simulink model "Vector_Control_Lib"  (R2021a)
settings: Solver=FixedStepDiscrete  StartTime=0.0  StopTime=1  FixedStep=Ts  RelTol=1e-3  EnableMultiTasking=on
values from neighbouring files (symbols this model uses):
  AccelTime = 1    [param.m]
  CurrentLSB = -1 * (1/ 0.1) * (3.3 / 2048)    (= -0.01611328125)    [param.m]
  DAC_ANALOG_MAX_0ch = 4    [param.m]
  DAC_ANALOG_MAX_1ch = 4    [param.m]
  DAC_PULSE_MAX = 4096    [param.m]
  DUTY_COUNTER_PERIOD_BASE = 2100    [param.m]
  EncoderLSB = 1/400    (= 0.0025)    [param.m]
  isEmbedded = swichSimulationMode('Emb')    [param.m]    (also in swichSimulationMode.m = boolean(0))
  Iu_ad_offset = 2020    [param.m]
  Iv_ad_offset = 2022    [param.m]
  Iw_ad_offset = 2020    [param.m]
  k_LPF = tauHPF / (tauHPF + Ts)    (= 0.999900009999)    [param.m]
  Ke = 4.50E-03    (= 0.0045)    [param.m]
  Ki_Ts = Ra / tauCurrent * Ts    (= 0.00075)    [param.m]
  Kp = La / tauCurrent    (= 0.009)    [param.m]
  La = 1.2e-3 * Ra    (= 0.0009)    [param.m]
  LockTime = 0.1    [param.m]
  omega_ref = 600    [param.m]
  Pn = 6    [param.m]
  Pz_ele = c2d(Ps_ele, Ts)    [param.m]
  Pz_mecha = c2d(Ps_mecha, Ts)    [param.m]
  TotalTime = LockTime + AccelTime    (= 1.1)    [param.m]
  Ts = 100e-6    (= 0.0001)    [param.m]
  Vdc = 10    [param.m]
libraries: simulink x21, arduinolib x4
settings Model: SILPILModeSetting=veronly  ExtModeTrigDuration=2  Creator=kuroda38  LastModifiedBy=kuroda38
settings OptimizationCC: EnhancedBackFolding=on  PassReuseOutputArgsAs=Individual arguments  ZeroExternalMemoryAtStartup=off  ZeroInternalMemoryAtStartup=off  MaxStackSize=64  OptimizeBlockOrder=speed  DifferentSizesBufferReuse=on  OptimizationCustomize=off  EfficientTunableParamExpr=on
settings DebuggingCC: ParameterTunabilityLossMsg=error
settings HardwareCC: ProdBitPerPointer=32  ProdBitPerSizeT=32  ProdBitPerPtrDiffT=32  ProdLargestAtomicInteger=Long  ProdLargestAtomicFloat=Double  ProdWordSize=32  ProdHWDeviceType=ARM Compatible->ARM Cortex  UseEmbeddedCoderFeatures=off  UseSimulinkCoderFeatures=off
settings SFSimCC: MATLABDynamicMemAlloc=off
settings RTWCC: SystemTargetFile=ert.tlc  HardwareBoard=Arduino Due  TemplateMakefile=ert_default_tmf  Toolchain=Arduino ARM  BuildConfiguration=Faster Runs
settings CodeAppCC: ForceParamTrailComments=on  IgnoreCustomStorageClasses=off  OperatorAnnotations=on  SimulinkDataObjDesc=on  SFDataObjDesc=on  InsertBlockDesc=on
settings ERTTargetCC: SupportContinuousTime=on  SupportNonInlinedSFcns=on  SupportVariableSizeSignals=on  ExtModeTransport=3  ExtModeStaticAlloc=on  ExtModeStaticAllocSize=24576  ExtModeMexFile=ext_xcp  ExtModeIntrfLevel=Level2 - Open

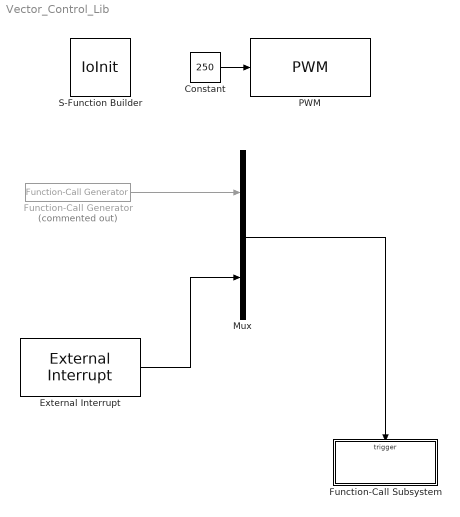
== system Vector_Control_Lib ==
  Constant : Constant  Value=250  OutDataTypeStr=uint8
  External Interrupt : arduinolib/External Interrupt  Pin=12  PullUp=off  Mode=RISING  InterruptSimulationInput=off
      settings: SourceProductBaseCode=ARDUINO
  Function-Call Generator : simulink/Ports & Subsystems/Function-Call Generator  Commented=on  sample_time=Ts  numberOfIterations=1  DisallowWideOutput=off
  Function-Call Subsystem : Subsystem  TreatAsAtomicUnit=on
  Mux : Mux  Inputs=2
  PWM : arduinolib/PWM  pinNumber=5  frequencyType=Specify  desiredFrequency=20000  achievableFrequency=20000
  S-Function Builder : S-Function  FunctionName=IoInit  SFunctionModules=IoInit_wrapper  SFunctionDeploymentMode=off  EnableBusSupport=off  mask(S-Function Builder){}
      mask help: Simulink:masks:SFunctionBuilder_MD
      mask init:
      | val = [[.9  0.75 0.75 1 1 .9 .9 1]',[1 1 0.75 0.75 .9 .9 1 .9]'];try , sys = get_param(gcb,'SfunBuilderFcnName');if isempty(sys), sys = get_param(gcb,'FunctionName'); end,catch, sys = get_param(gcb,'FunctionName'); end
      settings: CopyFcn=set_param(gcbh,'LinkStatus','none')  OpenFcn=sfunctionwizard(gcbh)
      mask Display:
      | plot(val(:,1),val(:,2))
      | disp(sys)
  wires:
  Constant/1 -> PWM/1
  Function-Call Generator/1 -> Mux/1
  Mux/1 -> Function-Call Subsystem/Trigger
  External Interrupt/1 -> Mux/2

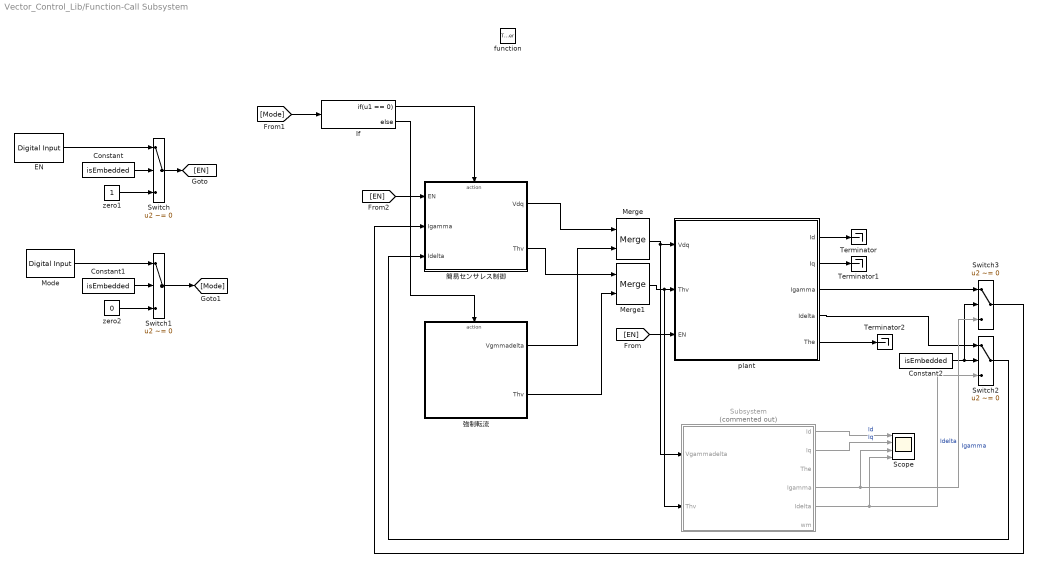
== system Vector_Control_Lib/Function-Call Subsystem ==
  function : TriggerPort  TriggerType=function-call  VariantControl=(inherit)
  Constant : Constant  Value=isEmbedded
  Constant1 : Constant  Value=isEmbedded
  Constant2 : Constant  Value=isEmbedded  OutDataTypeStr=uint8
  EN : arduinolib/Digital Input  pinNumber=7  mode=Default  Direction=input  SampleTime=-1  blockPlatform=arduino
  If : If  IfExpression=u1 == 0
  Merge : Merge
  Merge1 : Merge
  Mode : arduinolib/Digital Input  pinNumber=6  mode=Default  Direction=input  SampleTime=-1  blockPlatform=arduino
  Scope : Scope  NumInputPorts=4
  Subsystem : Subsystem  Commented=on
  Switch : Switch  Criteria=u2 ~= 0  OutDataTypeStr=uint16
  Switch1 : Switch  Criteria=u2 ~= 0  OutDataTypeStr=uint16
  Switch2 : Switch  Criteria=u2 ~= 0
  Switch3 : Switch  Criteria=u2 ~= 0
  Terminator : Terminator
  Terminator1 : Terminator
  Terminator2 : Terminator
  plant : Subsystem
  zero1 : Constant  OutDataTypeStr=uint16
  zero2 : Constant  Value=0  OutDataTypeStr=uint16
  強制転流 : Subsystem  TreatAsAtomicUnit=on
  簡易センサレス制御 : Subsystem  TreatAsAtomicUnit=on
  wires:
  [EN] -> plant/3(EN)
  Merge/1 -> plant/1(Vdq), Subsystem/1(Vgammadelta)
  Merge1/1 -> Subsystem/2(Thv), plant/2(Thv)
  If/1 -> 簡易センサレス制御/Action
  If/2 -> 強制転流/Action
  簡易センサレス制御/1(Vdq) -> Merge/1
  強制転流/1(Vgmmadelta) -> Merge/2
  簡易センサレス制御/2(Thv) -> Merge1/1
  強制転流/2(Thv) -> Merge1/2
  plant/1(Id) -> Terminator/1
  plant/2(Iq) -> Terminator1/1
  plant/5(The) -> Terminator2/1
  [EN] -> 簡易センサレス制御/1(EN)
  Constant/1 -> Switch/2
  Switch/1 -> [EN]
  EN/1 -> Switch/1
  zero1/1 -> Switch/3
  Constant1/1 -> Switch1/2
  zero2/1 -> Switch1/3
  Mode/1 -> Switch1/1
  Switch1/1 -> [Mode]
  [Mode] -> If/1
  Subsystem/1(Id) -> Scope/1  "Id"
  Subsystem/2(Iq) -> Scope/2  "Iq"
  plant/3(Igamma) -> Switch3/1
  plant/4(Idelta) -> Switch2/1
  Constant2/1 -> Switch3/2, Switch2/2
  Subsystem/4(Igamma) -> Scope/3, Switch3/3  "Igamma"
  Subsystem/5(Idelta) -> Scope/4, Switch2/3  "Idelta"
  Switch3/1 -> 簡易センサレス制御/2(Igamma)
  Switch2/1 -> 簡易センサレス制御/3(Idelta)

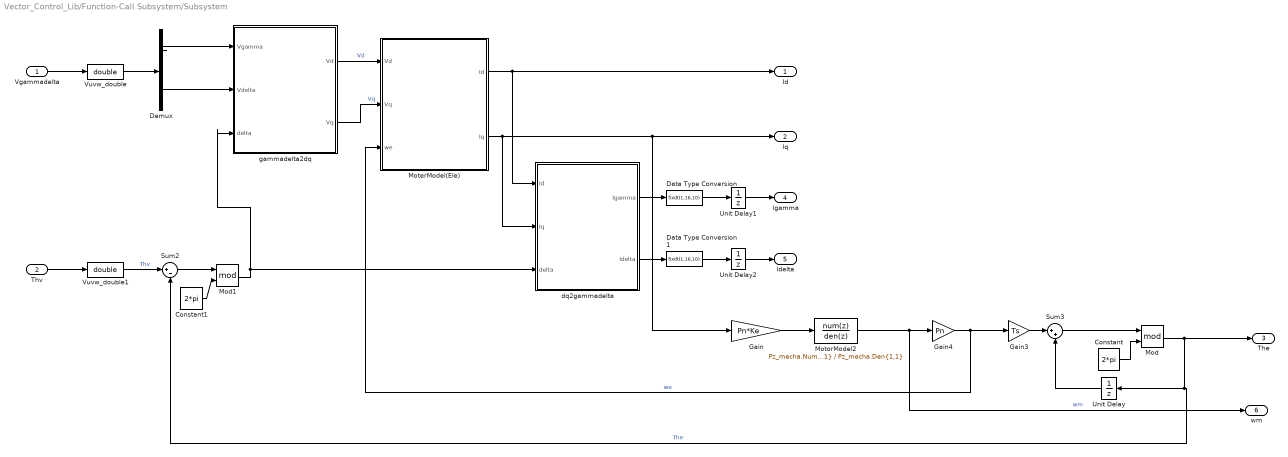
== system Vector_Control_Lib/Function-Call Subsystem/Subsystem ==
  Vgammadelta : Inport
  Thv : Inport  Port=2
  Constant : Constant  Value=2*pi
  Constant1 : Constant  Value=2*pi
  Data Type Conversion : DataTypeConversion  OutDataTypeStr=fixdt(1,16,10)
  Data Type Conversion1 : DataTypeConversion  OutDataTypeStr=fixdt(1,16,10)
  Demux : Demux  Outputs=2
  Gain : Gain  Gain=Pn*Ke
  Gain3 : Gain  Gain=Ts
  Gain4 : Gain  Gain=Pn
  Mod : Math  Operator=mod  SaturateOnIntegerOverflow=on
  Mod1 : Math  Operator=mod  SaturateOnIntegerOverflow=on
  MoterModel(Ele) : Subsystem
  MotorModel2 : DiscreteTransferFcn  Numerator=Pz_mecha.Num{1,1}  Denominator=Pz_mecha.Den{1,1}
  Sum2 : Sum  Inputs=|+-
  Sum3 : Sum  Inputs=|++
  Unit Delay : UnitDelay  SampleTime=-1  HasFrameUpgradeWarning=on
  Unit Delay1 : UnitDelay  SampleTime=-1  HasFrameUpgradeWarning=on
  Unit Delay2 : UnitDelay  SampleTime=-1  HasFrameUpgradeWarning=on
  Vuvw_double : DataTypeConversion  OutDataTypeStr=double
  Vuvw_double1 : DataTypeConversion  OutDataTypeStr=double
  dq2gammadelta : Subsystem
  gammadelta2dq : Subsystem
  Id : Outport
  Iq : Outport  Port=2
  The : Outport  Port=3
  Igamma : Outport  Port=4
  Idelta : Outport  Port=5
  wm : Outport  Port=6
  wires:
  Gain/1 -> MotorModel2/1
  MotorModel2/1 -> wm/1, Gain4/1  "wm"
  Vgammadelta/1 -> Vuvw_double/1
  Gain3/1 -> Sum3/1
  Vuvw_double/1 -> Demux/1
  Thv/1 -> Vuvw_double1/1
  Gain4/1 -> MoterModel(Ele)/3(we), Gain3/1  "we"
  Demux/1 -> gammadelta2dq/1(Vgamma)
  Demux/2 -> gammadelta2dq/2(Vdelta)
  MoterModel(Ele)/2(Iq) -> dq2gammadelta/2(Iq), Gain/1, Iq/1
  gammadelta2dq/1(Vd) -> MoterModel(Ele)/1(Vd)  "Vd"
  gammadelta2dq/2(Vq) -> MoterModel(Ele)/2(Vq)  "Vq"
  MoterModel(Ele)/1(Id) -> dq2gammadelta/1(Id), Id/1
  dq2gammadelta/1(Igamma) -> Data Type Conversion/1
  dq2gammadelta/2(Idelta) -> Data Type Conversion1/1
  Vuvw_double1/1 -> Sum2/1  "Thv"
  Constant/1 -> Mod/2
  Sum3/1 -> Mod/1
  Mod/1 -> Unit Delay/1, Sum2/2, The/1  "The"
  Unit Delay/1 -> Sum3/2
  Constant1/1 -> Mod1/2
  Sum2/1 -> Mod1/1
  Mod1/1 -> dq2gammadelta/3(delta), gammadelta2dq/3(delta)
  Data Type Conversion/1 -> Unit Delay1/1
  Unit Delay1/1 -> Igamma/1
  Data Type Conversion1/1 -> Unit Delay2/1
  Unit Delay2/1 -> Idelta/1

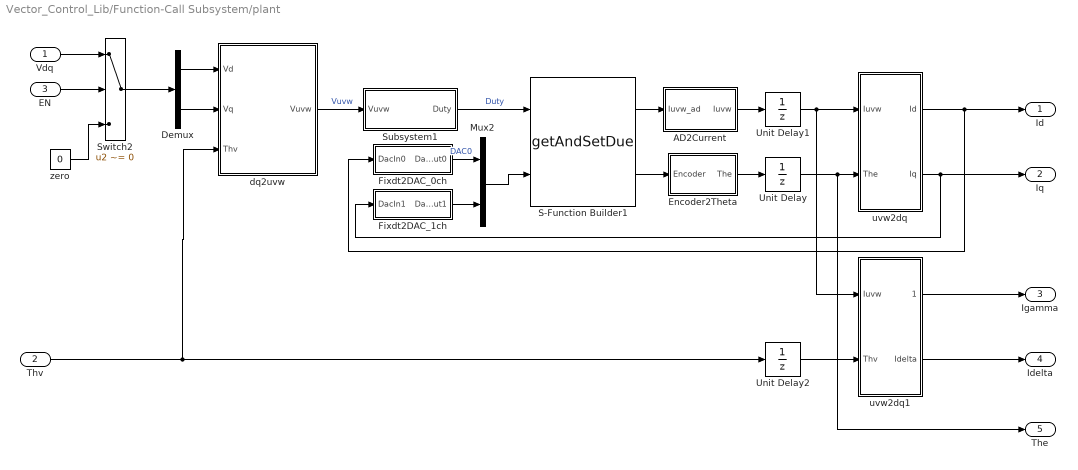
== system Vector_Control_Lib/Function-Call Subsystem/plant ==
  Vdq : Inport
  Thv : Inport  Port=2
  EN : Inport  Port=3
  AD2Current : Subsystem
  Demux : Demux  Outputs=2
  Encoder2Theta : Subsystem
  Fixdt2DAC_0ch : Subsystem
  Fixdt2DAC_1ch : Subsystem
  Mux2 : Mux  Inputs=2
  S-Function Builder1 : S-Function  FunctionName=getAndSetDue  SFunctionModules=getAndSetDue_wrapper  SFunctionDeploymentMode=off  EnableBusSupport=off  mask(S-Function Builder){}
      mask help: Simulink:masks:SFunctionBuilder_MD
      mask init: same as Vector_Control_Lib/S-Function Builder
      settings: CopyFcn=set_param(gcbh,'LinkStatus','none')  OpenFcn=sfunctionwizard(gcbh)
      mask Display:
      | plot(val(:,1),val(:,2))
      | disp(sys)
      | port_label('input',1,'Duty')
      | port_label('input',2,'DAC')
      | port_label('output',1,'Iuvw')
      | port_label('output',2,'Encoder')
  Subsystem1 : Subsystem
  Switch2 : Switch  Criteria=u2 ~= 0  OutDataTypeStr=fixdt(1,16,10)
  Unit Delay : UnitDelay  SampleTime=-1  HasFrameUpgradeWarning=on
  Unit Delay1 : UnitDelay  SampleTime=-1  HasFrameUpgradeWarning=on
  Unit Delay2 : UnitDelay  SampleTime=-1  HasFrameUpgradeWarning=on
  dq2uvw : Subsystem
  uvw2dq : Subsystem
  uvw2dq1 : Subsystem
  zero : Constant  Value=0  OutDataTypeStr=fixdt(1,16,10)
  Id : Outport
  Iq : Outport  Port=2
  Igamma : Outport  Port=3
  Idelta : Outport  Port=4
  The : Outport  Port=5
  wires:
  S-Function Builder1/2 -> Encoder2Theta/1(Encoder)
  AD2Current/1(Iuvw) -> Unit Delay1/1
  uvw2dq/2(Iq) -> Fixdt2DAC_1ch/1(DacIn1), Iq/1
  Fixdt2DAC_1ch/1(DacOut1) -> Mux2/2
  Fixdt2DAC_0ch/1(DacOut0) -> Mux2/1  "DAC0"
  Mux2/1 -> S-Function Builder1/2
  uvw2dq/1(Id) -> Id/1, Fixdt2DAC_0ch/1(DacIn0)
  Unit Delay/1 -> The/1, uvw2dq/2(The)
  dq2uvw/1(Vuvw) -> Subsystem1/1(Vuvw)  "Vuvw"
  Subsystem1/1(Duty) -> S-Function Builder1/1  "Duty"
  S-Function Builder1/1 -> AD2Current/1(Iuvw_ad)
  Unit Delay1/1 -> uvw2dq1/1(Iuvw), uvw2dq/1(Iuvw)
  Encoder2Theta/1(The) -> Unit Delay/1
  Thv/1 -> dq2uvw/3(Thv), Unit Delay2/1
  Vdq/1 -> Switch2/1
  EN/1 -> Switch2/2
  zero/1 -> Switch2/3
  Switch2/1 -> Demux/1
  Demux/1 -> dq2uvw/1(Vd)
  Demux/2 -> dq2uvw/2(Vq)
  uvw2dq1/1(Igamma) -> Igamma/1
  uvw2dq1/2(Idelta) -> Idelta/1
  Unit Delay2/1 -> uvw2dq1/2(Thv)

== system Vector_Control_Lib/Function-Call Subsystem/強制転流 ==
  Action Port : ActionPort  ActionPortLabel=else
  Mux : Mux  Inputs=2
  Omega_ref : Constant  Value=omega_ref  OutDataTypeStr=fixedTypeOmegaRef
  Vdelta : Constant  Value=2  OutDataTypeStr=fixdt(1,16,10)
  Vgamma : Constant  Value=0  OutDataTypeStr=fixdt(1,16,10)
  wv_integral : Subsystem
  Vgmmadelta : Outport
  Thv : Outport  Port=2
  wires:
  Vgamma/1 -> Mux/1
  Vdelta/1 -> Mux/2
  Mux/1 -> Vgmmadelta/1
  Omega_ref/1 -> wv_integral/1(wv_ref)  "Omega_ref"
  wv_integral/1(Thv) -> Thv/1  "Thv"

== system Vector_Control_Lib/Function-Call Subsystem/簡易センサレス制御 ==
  EN : Inport
  Igamma : Inport  Port=2
  Idelta : Inport  Port=3
  Action Port : ActionPort  ActionPortLabel=if(u1 == 0)
  Mux : Mux  Inputs=2
  VdeltaController : Subsystem
  Vgamma : Constant  Value=0  OutDataTypeStr=fixdt(1,16,10)
  wv_integral : Subsystem
  Vdq : Outport
  Thv : Outport  Port=2
  wires:
  Mux/1 -> Vdq/1
  EN/1 -> VdeltaController/1(EN)
  wv_integral/1(Thv) -> Thv/1  "Thv"
  VdeltaController/1(Omega_ref) -> wv_integral/1(wv_ref)  "Omega_ref"
  Vgamma/1 -> Mux/1
  Igamma/1 -> VdeltaController/2(Igamma)
  Idelta/1 -> VdeltaController/3(Idelta)
  VdeltaController/2(Vdelta) -> Mux/2

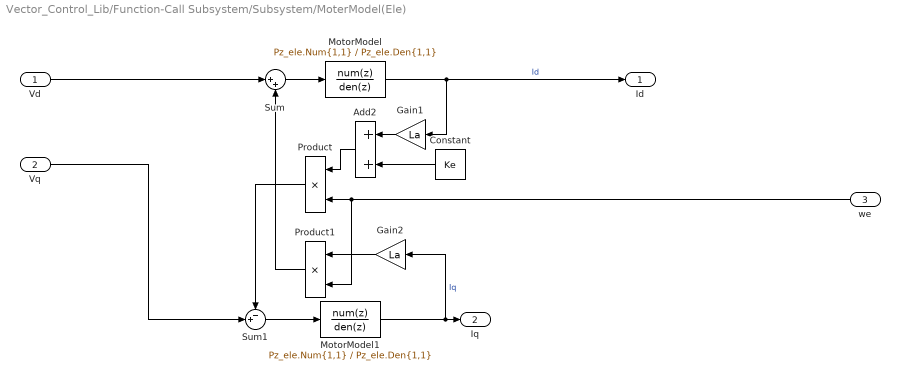
== system Vector_Control_Lib/Function-Call Subsystem/Subsystem/MoterModel(Ele) ==
  Vd : Inport
  Vq : Inport  Port=2
  we : Inport  Port=3
  Add2 : Sum
  Constant : Constant  Value=Ke
  Gain1 : Gain  Gain=La
  Gain2 : Gain  Gain=La
  MotorModel : DiscreteTransferFcn  Numerator=Pz_ele.Num{1,1}  Denominator=Pz_ele.Den{1,1}
  MotorModel1 : DiscreteTransferFcn  Numerator=Pz_ele.Num{1,1}  Denominator=Pz_ele.Den{1,1}
  Product : Product
  Product1 : Product
  Sum : Sum  Inputs=|++
  Sum1 : Sum  Inputs=-+|
  Id : Outport
  Iq : Outport  Port=2
  wires:
  we/1 -> Product1/2, Product/2
  MotorModel/1 -> Id/1, Gain1/1  "Id"
  Gain2/1 -> Product1/1
  Product/1 -> Sum1/1
  Constant/1 -> Add2/2
  Sum/1 -> MotorModel/1
  Gain1/1 -> Add2/1
  Product1/1 -> Sum/2
  Sum1/1 -> MotorModel1/1
  Add2/1 -> Product/1
  Vd/1 -> Sum/1
  Vq/1 -> Sum1/2
  MotorModel1/1 -> Gain2/1, Iq/1  "Iq"

== system Vector_Control_Lib/Function-Call Subsystem/Subsystem/dq2gammadelta ==
  Id : Inport
  Iq : Inport  Port=2
  delta : Inport  Port=3
  Add : Sum
  Add1 : Sum  Inputs=-+
  Cos2 : Trigonometry
  Cos3 : Trigonometry  Operator=cos
  Product{2..5} (4 alike) : Product
  Igamma : Outport
  Idelta : Outport  Port=2
  wires:
  delta/1 -> Cos2/1, Cos3/1
  Iq/1 -> Product5/1, Product3/1
  Product4/1 -> Add1/1
  Cos3/1 -> Product5/2, Product2/2
  Product3/1 -> Add/2
  Id/1 -> Product4/1, Product2/1
  Product2/1 -> Add/1
  Product5/1 -> Add1/2
  Cos2/1 -> Product3/2, Product4/2
  Add1/1 -> Idelta/1
  Add/1 -> Igamma/1

== system Vector_Control_Lib/Function-Call Subsystem/Subsystem/gammadelta2dq ==
  Vgamma : Inport
  Vdelta : Inport  Port=2
  delta : Inport  Port=3
  Add : Sum  Inputs=+-
  Add1 : Sum
  Cos2 : Trigonometry
  Cos3 : Trigonometry  Operator=cos
  Product{2..5} (4 alike) : Product
  Vd : Outport
  Vq : Outport  Port=2
  wires:
  delta/1 -> Cos2/1, Cos3/1
  Vdelta/1 -> Product5/1, Product3/1
  Product4/1 -> Add1/1
  Cos3/1 -> Product5/2, Product2/2
  Product3/1 -> Add/2
  Vgamma/1 -> Product4/1, Product2/1
  Product2/1 -> Add/1
  Product5/1 -> Add1/2
  Cos2/1 -> Product3/2, Product4/2
  Add1/1 -> Vq/1
  Add/1 -> Vd/1

== system Vector_Control_Lib/Function-Call Subsystem/plant/AD2Current ==
  Iuvw_ad : Inport
  Add : Sum  Inputs=+-  OutDataTypeStr=int16
  Add1 : Sum  Inputs=+-  OutDataTypeStr=int16
  Add2 : Sum  Inputs=+-  OutDataTypeStr=int16
  Constant : Constant  Value=Iu_ad_offset  OutDataTypeStr=uint16
  Constant1 : Constant  Value=Iv_ad_offset  OutDataTypeStr=uint16
  Constant2 : Constant  Value=CurrentLSB  OutDataTypeStr=fixdt(1,16)
  Constant3 : Constant  Value=Iw_ad_offset  OutDataTypeStr=uint16
  Demux : Demux  Outputs=3
  Mux : Mux  Inputs=3
  Product : Product  OutDataTypeStr=fixedTypeDqCurrent
  Iuvw : Outport
  wires:
  Demux/2 -> Add1/1
  Constant/1 -> Add/2
  Constant3/1 -> Add2/2
  Demux/3 -> Add2/1
  Constant1/1 -> Add1/2
  Demux/1 -> Add/1
  Add/1 -> Mux/1
  Add1/1 -> Mux/2
  Add2/1 -> Mux/3
  Product/1 -> Iuvw/1
  Constant2/1 -> Product/2
  Mux/1 -> Product/1
  Iuvw_ad/1 -> Demux/1

== system Vector_Control_Lib/Function-Call Subsystem/plant/Encoder2Theta ==
  Encoder : Inport
  Add : Sum  Inputs=+-  OutDataTypeStr=int16
  Constant : Constant  Value=36  OutDataTypeStr=uint16
  Constant1 : Constant  Value=EncoderLSB  OutDataTypeStr=fixedTypeMaxOne
  Constant2 : Constant  Value=Pn  OutDataTypeStr=ufixedTypeMaxTwenty
  Constant3 : Constant  Value=2*pi  OutDataTypeStr=ufixedTypeTwoPi
  Product : Product  OutDataTypeStr=ufixedTypeMaxOne
  Product1 : Product  OutDataTypeStr=fixdt(0,16,16)
  Product7 : Product  OutDataTypeStr=ufixedTypeTwoPi
  The : Outport
  wires:
  Encoder/1 -> Add/1
  Constant/1 -> Add/2
  Add/1 -> Product/1
  Constant1/1 -> Product/2
  Product/1 -> Product1/1
  Constant2/1 -> Product1/2
  Product1/1 -> Product7/1
  Product7/1 -> The/1
  Constant3/1 -> Product7/2

== system Vector_Control_Lib/Function-Call Subsystem/plant/Fixdt2DAC_0ch ==
  DacIn0 : Inport
  Add1 : Sum  OutDataTypeStr=fixdt(1,16,10)
  Constant4 : Constant  Value=DAC_ANALOG_MAX_0ch  OutDataTypeStr=fixdt(1,16)
  Constant7 : Constant  Value=(DAC_PULSE_MAX / 2 ) / DAC_ANALOG_MAX_0ch  OutDataTypeStr=fixdt(1,16)  LockScale=on
  Product1 : Product  OutDataTypeStr=uint16
  DacOut0 : Outport
  wires:
  Add1/1 -> Product1/1
  Constant7/1 -> Product1/2
  Constant4/1 -> Add1/2
  Product1/1 -> DacOut0/1
  DacIn0/1 -> Add1/1

== system Vector_Control_Lib/Function-Call Subsystem/plant/Fixdt2DAC_1ch ==
  DacIn1 : Inport
  Add1 : Sum  OutDataTypeStr=fixdt(1,16,10)
  Constant4 : Constant  Value=DAC_ANALOG_MAX_1ch  OutDataTypeStr=fixdt(1,16)
  Constant7 : Constant  Value=(DAC_PULSE_MAX / 2 ) / DAC_ANALOG_MAX_1ch  OutDataTypeStr=fixdt(1,16)  LockScale=on
  Product1 : Product  OutDataTypeStr=uint16
  DacOut1 : Outport
  wires:
  Add1/1 -> Product1/1
  Constant7/1 -> Product1/2
  Constant4/1 -> Add1/2
  Product1/1 -> DacOut1/1
  DacIn1/1 -> Add1/1

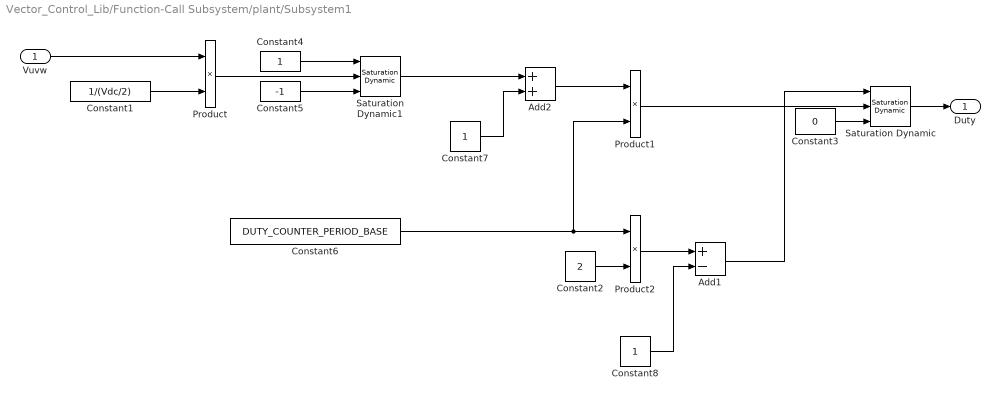
== system Vector_Control_Lib/Function-Call Subsystem/plant/Subsystem1 ==
  Vuvw : Inport
  Add1 : Sum  Inputs=+-  OutDataTypeStr=uint16
  Add2 : Sum  OutDataTypeStr=ufixedTypeMaxOne
  Constant1 : Constant  Value=1/(Vdc/2)  OutDataTypeStr=fixdt(1,16)
  Constant2 : Constant  Value=2  OutDataTypeStr=uint16
  Constant3 : Constant  Value=0  OutDataTypeStr=Inherit: Inherit via back propagation
  Constant4 : Constant  OutDataTypeStr=fixedTypeMaxOne
  Constant5 : Constant  Value=-1  OutDataTypeStr=fixedTypeMaxOne
  Constant6 : Constant  Value=DUTY_COUNTER_PERIOD_BASE  OutDataTypeStr=uint16
  Constant7 : Constant  OutDataTypeStr=fixedTypeMaxOne
  Constant8 : Constant  OutDataTypeStr=uint16
  Product : Product  OutDataTypeStr=fixedTypeMaxOne
  Product1 : Product
  Product2 : Product  OutDataTypeStr=uint16
  Saturation Dynamic : simulink/Discontinuities/Saturation Dynamic  OutMin=[]  OutMax=[]  OutDataTypeStr=fixdt(0,16,0)  OutputDataTypeScalingMode=Specify via dialog  OutDataType=fixdt(0,16,0)  OutScaling=[]  DoSatur=off
  Saturation Dynamic1 : simulink/Discontinuities/Saturation Dynamic  OutMin=[]  OutMax=[]  OutDataTypeStr=fixedTypeMaxOne  OutputDataTypeScalingMode=Specify via dialog  OutDataType=fixedTypeMaxOne  OutScaling=[]  DoSatur=off
  Duty : Outport
  wires:
  Constant7/1 -> Add2/2
  Constant1/1 -> Product/2
  Product/1 -> Saturation Dynamic1/2
  Saturation Dynamic1/1 -> Add2/1
  Product1/1 -> Saturation Dynamic/2
  Saturation Dynamic/1 -> Duty/1
  Add2/1 -> Product1/1
  Vuvw/1 -> Product/1
  Add1/1 -> Saturation Dynamic/1
  Constant3/1 -> Saturation Dynamic/3
  Constant4/1 -> Saturation Dynamic1/1
  Constant5/1 -> Saturation Dynamic1/3
  Product2/1 -> Add1/1
  Constant8/1 -> Add1/2
  Constant2/1 -> Product2/2
  Constant6/1 -> Product1/2, Product2/1

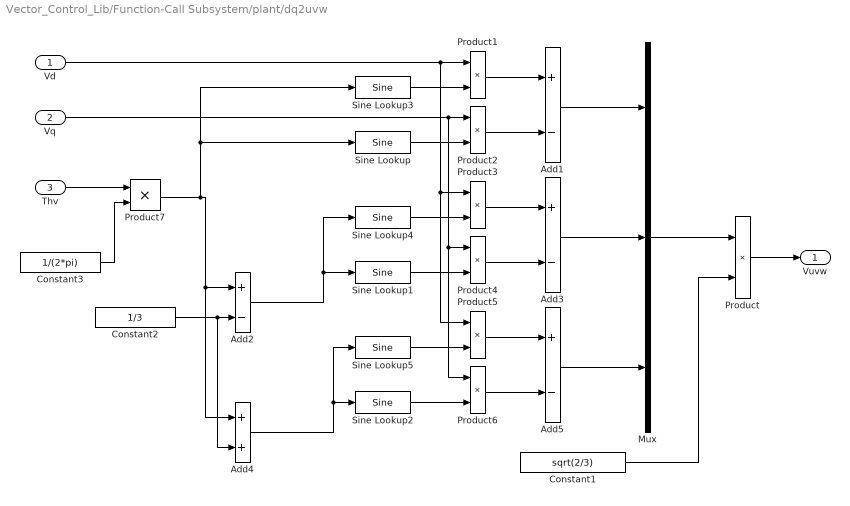
== system Vector_Control_Lib/Function-Call Subsystem/plant/dq2uvw ==
  Vd : Inport
  Vq : Inport  Port=2
  Thv : Inport  Port=3
  Add1 : Sum  Inputs=+-
  Add2 : Sum  Inputs=+-  OutDataTypeStr=fixedTypeMaxOne
  Add3 : Sum  Inputs=+-
  Add4 : Sum  OutDataTypeStr=fixedTypeMaxOne
  Add5 : Sum  Inputs=+-
  Constant1 : Constant  Value=sqrt(2/3)  OutDataTypeStr=fixdt(1,16)
  Constant2 : Constant  Value=1/3  OutDataTypeStr=fixdt(1,16)
  Constant3 : Constant  Value=1/(2*pi)  OutDataTypeStr=fixdt(1,16)
  Mux : Mux  Inputs=3
  Product{,1..6} (7 alike) : Product  OutDataTypeStr=fixedTypeDqVoltage
  Product7 : Product  OutDataTypeStr=fixedTypeMaxOne
  Sine Lookup : simulink/Lookup Tables/Sine  Formula=sin(2*pi*u)  NumDataPoints=(2^5)+1  OutputWordLength=16  InternalRulePriority=Speed
  Sine Lookup1 : simulink/Lookup Tables/Sine  Formula=sin(2*pi*u)  NumDataPoints=(2^5)+1  OutputWordLength=16  InternalRulePriority=Speed
  Sine Lookup2 : simulink/Lookup Tables/Sine  Formula=sin(2*pi*u)  NumDataPoints=(2^5)+1  OutputWordLength=16  InternalRulePriority=Speed
  Sine Lookup3 : simulink/Lookup Tables/Sine  Formula=cos(2*pi*u)  NumDataPoints=(2^5)+1  OutputWordLength=16  InternalRulePriority=Speed
  Sine Lookup4 : simulink/Lookup Tables/Sine  Formula=cos(2*pi*u)  NumDataPoints=(2^5)+1  OutputWordLength=16  InternalRulePriority=Speed
  Sine Lookup5 : simulink/Lookup Tables/Sine  Formula=cos(2*pi*u)  NumDataPoints=(2^5)+1  OutputWordLength=16  InternalRulePriority=Speed
  Vuvw : Outport
  wires:
  Vq/1 -> Product2/1, Product6/1, Product4/1
  Vd/1 -> Product1/1, Product5/1, Product3/1
  Sine Lookup/1 -> Product2/2
  Product1/1 -> Add1/1
  Sine Lookup3/1 -> Product1/2
  Product2/1 -> Add1/2
  Add1/1 -> Mux/1
  Mux/1 -> Product/1
  Constant1/1 -> Product/2
  Product/1 -> Vuvw/1
  Add3/1 -> Mux/2
  Sine Lookup1/1 -> Product4/2
  Product4/1 -> Add3/2
  Product3/1 -> Add3/1
  Add2/1 -> Sine Lookup4/1, Sine Lookup1/1
  Sine Lookup4/1 -> Product3/2
  Product6/1 -> Add5/2
  Sine Lookup5/1 -> Product5/2
  Product5/1 -> Add5/1
  Add4/1 -> Sine Lookup5/1, Sine Lookup2/1
  Sine Lookup2/1 -> Product6/2
  Add5/1 -> Mux/3
  Constant2/1 -> Add4/2, Add2/2
  Product7/1 -> Add4/1, Add2/1, Sine Lookup3/1, Sine Lookup/1
  Thv/1 -> Product7/1
  Constant3/1 -> Product7/2

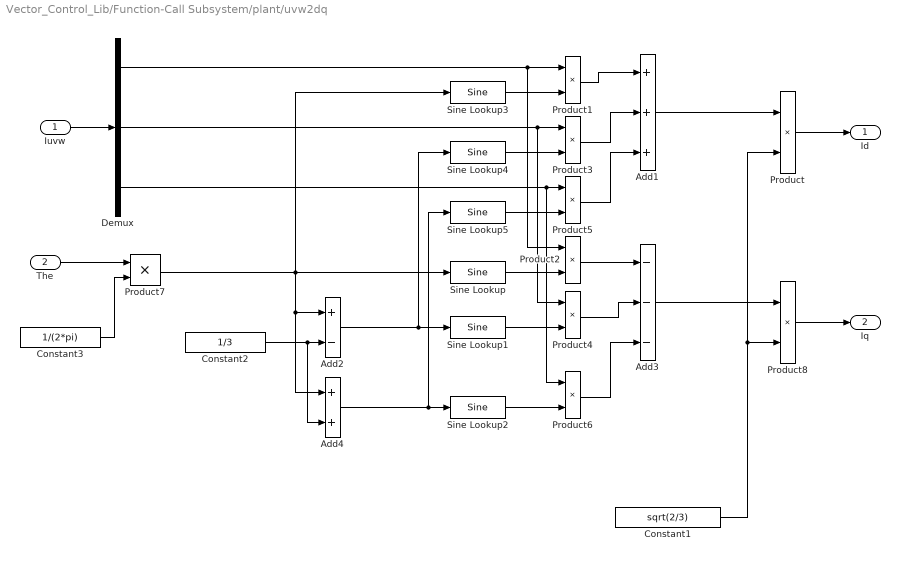
== system Vector_Control_Lib/Function-Call Subsystem/plant/uvw2dq ==
  Iuvw : Inport
  The : Inport  Port=2
  Add1 : Sum  Inputs=+++
  Add2 : Sum  Inputs=+-  OutDataTypeStr=fixedTypeMaxOne
  Add3 : Sum  Inputs=---
  Add4 : Sum  OutDataTypeStr=fixedTypeMaxOne
  Constant1 : Constant  Value=sqrt(2/3)  OutDataTypeStr=fixdt(1,16,14)
  Constant2 : Constant  Value=1/3  OutDataTypeStr=fixdt(1,16)
  Constant3 : Constant  Value=1/(2*pi)  OutDataTypeStr=fixdt(1,16)
  Demux : Demux  Outputs=3
  Product{,1..6,8} (8 alike) : Product  OutDataTypeStr=fixedTypeDqCurrent
  Product7 : Product  OutDataTypeStr=fixedTypeMaxOne
  Sine Lookup : simulink/Lookup Tables/Sine  Formula=sin(2*pi*u)  NumDataPoints=(2^5)+1  OutputWordLength=16  InternalRulePriority=Speed
  Sine Lookup1 : simulink/Lookup Tables/Sine  Formula=sin(2*pi*u)  NumDataPoints=(2^5)+1  OutputWordLength=16  InternalRulePriority=Speed
  Sine Lookup2 : simulink/Lookup Tables/Sine  Formula=sin(2*pi*u)  NumDataPoints=(2^5)+1  OutputWordLength=16  InternalRulePriority=Speed
  Sine Lookup3 : simulink/Lookup Tables/Sine  Formula=cos(2*pi*u)  NumDataPoints=(2^5)+1  OutputWordLength=16  InternalRulePriority=Speed
  Sine Lookup4 : simulink/Lookup Tables/Sine  Formula=cos(2*pi*u)  NumDataPoints=(2^5)+1  OutputWordLength=16  InternalRulePriority=Speed
  Sine Lookup5 : simulink/Lookup Tables/Sine  Formula=cos(2*pi*u)  NumDataPoints=(2^5)+1  OutputWordLength=16  InternalRulePriority=Speed
  Id : Outport
  Iq : Outport  Port=2
  wires:
  Constant3/1 -> Product7/2
  The/1 -> Product7/1
  Sine Lookup4/1 -> Product3/2
  Sine Lookup2/1 -> Product6/2
  Sine Lookup/1 -> Product2/2
  Product6/1 -> Add3/3
  Product7/1 -> Sine Lookup3/1, Add4/1, Add2/1, Sine Lookup/1
  Sine Lookup3/1 -> Product1/2
  Add2/1 -> Sine Lookup4/1, Sine Lookup1/1
  Sine Lookup5/1 -> Product5/2
  Constant1/1 -> Product8/2, Product/2
  Sine Lookup1/1 -> Product4/2
  Product/1 -> Id/1
  Constant2/1 -> Add4/2, Add2/2
  Product1/1 -> Add1/1
  Add4/1 -> Sine Lookup5/1, Sine Lookup2/1
  Iuvw/1 -> Demux/1
  Product3/1 -> Add1/2
  Product5/1 -> Add1/3
  Product2/1 -> Add3/1
  Product4/1 -> Add3/2
  Demux/1 -> Product2/1, Product1/1
  Demux/2 -> Product4/1, Product3/1
  Demux/3 -> Product6/1, Product5/1
  Add1/1 -> Product/1
  Add3/1 -> Product8/1
  Product8/1 -> Iq/1

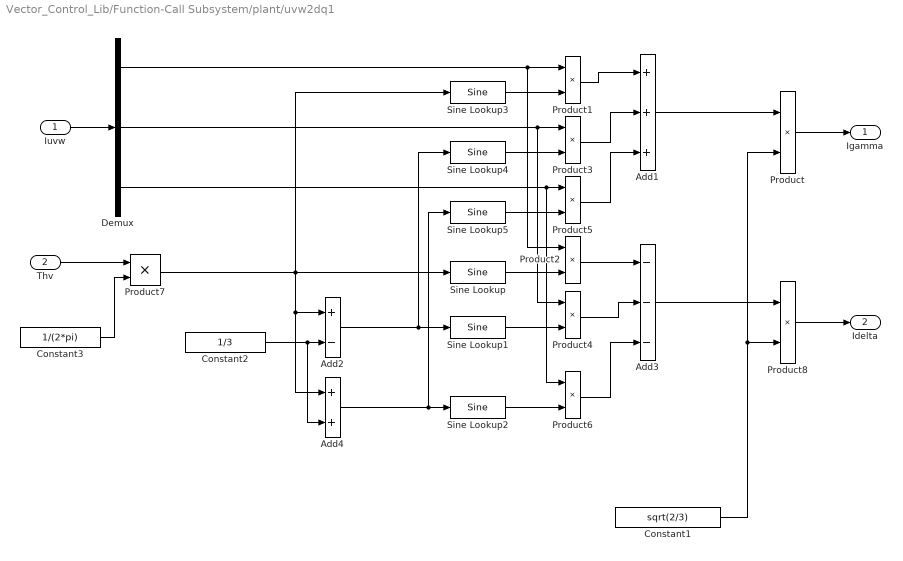
== system Vector_Control_Lib/Function-Call Subsystem/plant/uvw2dq1 ==
  Iuvw : Inport
  Thv : Inport  Port=2
  Add1 : Sum  Inputs=+++
  Add2 : Sum  Inputs=+-  OutDataTypeStr=fixedTypeMaxOne
  Add3 : Sum  Inputs=---
  Add4 : Sum  OutDataTypeStr=fixedTypeMaxOne
  Constant1 : Constant  Value=sqrt(2/3)  OutDataTypeStr=fixdt(1,16,14)
  Constant2 : Constant  Value=1/3  OutDataTypeStr=fixdt(1,16)
  Constant3 : Constant  Value=1/(2*pi)  OutDataTypeStr=fixdt(1,16)
  Demux : Demux  Outputs=3
  Product{,1..6,8} (8 alike) : Product  OutDataTypeStr=fixedTypeDqCurrent
  Product7 : Product  OutDataTypeStr=fixedTypeMaxOne
  Sine Lookup : simulink/Lookup Tables/Sine  Formula=sin(2*pi*u)  NumDataPoints=(2^5)+1  OutputWordLength=16  InternalRulePriority=Speed
  Sine Lookup1 : simulink/Lookup Tables/Sine  Formula=sin(2*pi*u)  NumDataPoints=(2^5)+1  OutputWordLength=16  InternalRulePriority=Speed
  Sine Lookup2 : simulink/Lookup Tables/Sine  Formula=sin(2*pi*u)  NumDataPoints=(2^5)+1  OutputWordLength=16  InternalRulePriority=Speed
  Sine Lookup3 : simulink/Lookup Tables/Sine  Formula=cos(2*pi*u)  NumDataPoints=(2^5)+1  OutputWordLength=16  InternalRulePriority=Speed
  Sine Lookup4 : simulink/Lookup Tables/Sine  Formula=cos(2*pi*u)  NumDataPoints=(2^5)+1  OutputWordLength=16  InternalRulePriority=Speed
  Sine Lookup5 : simulink/Lookup Tables/Sine  Formula=cos(2*pi*u)  NumDataPoints=(2^5)+1  OutputWordLength=16  InternalRulePriority=Speed
  Igamma : Outport
  Idelta : Outport  Port=2
  wires:
  Product8/1 -> Idelta/1
  Add3/1 -> Product8/1
  Add1/1 -> Product/1
  Demux/3 -> Product5/1, Product6/1
  Demux/2 -> Product3/1, Product4/1
  Demux/1 -> Product1/1, Product2/1
  Product4/1 -> Add3/2
  Product2/1 -> Add3/1
  Product5/1 -> Add1/3
  Product3/1 -> Add1/2
  Iuvw/1 -> Demux/1
  Add4/1 -> Sine Lookup2/1, Sine Lookup5/1
  Product1/1 -> Add1/1
  Constant2/1 -> Add2/2, Add4/2
  Product/1 -> Igamma/1
  Sine Lookup1/1 -> Product4/2
  Constant1/1 -> Product/2, Product8/2
  Sine Lookup5/1 -> Product5/2
  Add2/1 -> Sine Lookup1/1, Sine Lookup4/1
  Sine Lookup3/1 -> Product1/2
  Product7/1 -> Sine Lookup/1, Add2/1, Add4/1, Sine Lookup3/1
  Product6/1 -> Add3/3
  Sine Lookup/1 -> Product2/2
  Sine Lookup2/1 -> Product6/2
  Sine Lookup4/1 -> Product3/2
  Thv/1 -> Product7/1
  Constant3/1 -> Product7/2

== system Vector_Control_Lib/Function-Call Subsystem/強制転流/wv_integral ==
  wv_ref : Inport
  Constant : Constant  Value=2*pi  OutDataTypeStr=ufixedTypeTwoPi
  Constant1 : Constant  Value=Ts  OutDataTypeStr=fixdt(0,16)
  Constant3 : Constant  Value=0  OutDataTypeStr=fixdt(1,16)
  Product : Product  OutDataTypeStr=fixdt(0,16,10)
  Relational Operator : RelationalOperator  Operator=<  OutDataTypeStr=boolean  RndMeth=Simplest
  Sum : Sum  Inputs=|++  OutDataTypeStr=ufixedTypeTwoPi
  Switch : Switch  Criteria=u2 ~= 0  OutDataTypeStr=ufixedTypeTwoPi
  Unit Delay : UnitDelay  SampleTime=-1  HasFrameUpgradeWarning=on
  Thv : Outport
  wires:
  Product/1 -> Sum/1
  wv_ref/1 -> Product/1
  Relational Operator/1 -> Switch/2
  Sum/1 -> Switch/1, Relational Operator/1
  Constant/1 -> Relational Operator/2
  Switch/1 -> Thv/1, Unit Delay/1
  Unit Delay/1 -> Sum/2
  Constant3/1 -> Switch/3
  Constant1/1 -> Product/2

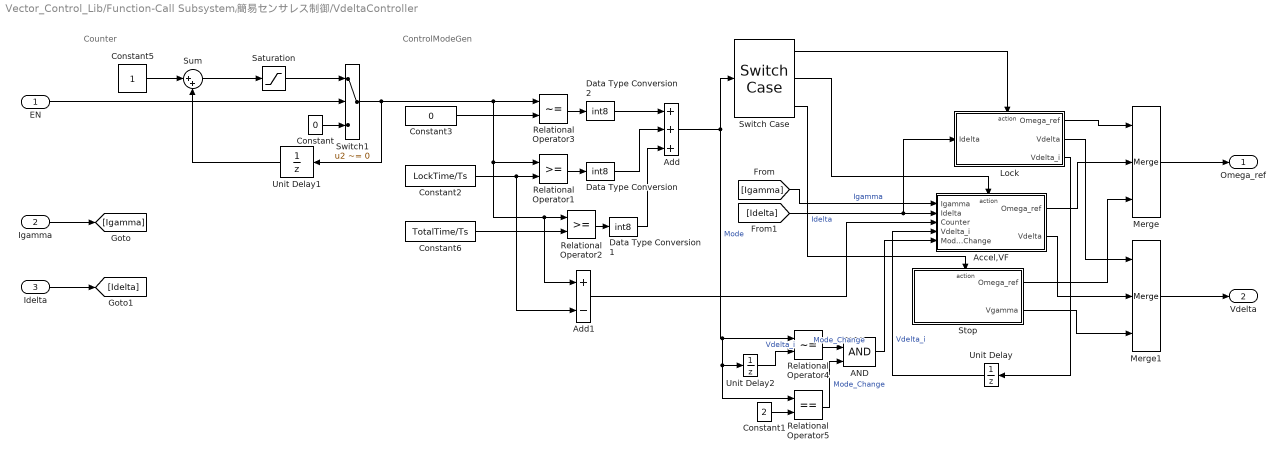
== system Vector_Control_Lib/Function-Call Subsystem/簡易センサレス制御/VdeltaController ==
  note: ControlModeGen
  note: Counter
  EN : Inport
  Igamma : Inport  Port=2
  Idelta : Inport  Port=3
  AND : Logic  IconShape=distinctive  AllPortsSameDT=off  OutDataTypeStr=boolean
  Accel,VF : Subsystem  TreatAsAtomicUnit=on
  Add : Sum  Inputs=+++
  Add1 : Sum  Inputs=+-  OutDataTypeStr=uint16
  Constant : Constant  Value=0  OutDataTypeStr=uint16
  Constant1 : Constant  Value=2  OutDataTypeStr=uint8
  Constant2 : Constant  Value=LockTime/Ts  OutDataTypeStr=uint16
  Constant3 : Constant  Value=0  OutDataTypeStr=uint16
  Constant5 : Constant  OutDataTypeStr=uint16
  Constant6 : Constant  Value=TotalTime/Ts  OutDataTypeStr=uint16
  Data Type Conversion : DataTypeConversion  OutDataTypeStr=int8
  Data Type Conversion1 : DataTypeConversion  OutDataTypeStr=int8
  Data Type Conversion2 : DataTypeConversion  OutDataTypeStr=int8
  Lock : Subsystem  TreatAsAtomicUnit=on
  Merge : Merge  Inputs=3
  Merge1 : Merge  Inputs=3
  Relational Operator1 : RelationalOperator  OutDataTypeStr=boolean  RndMeth=Simplest
  Relational Operator2 : RelationalOperator  OutDataTypeStr=boolean  RndMeth=Simplest
  Relational Operator3 : RelationalOperator  Operator=~=  OutDataTypeStr=boolean  RndMeth=Simplest
  Relational Operator4 : RelationalOperator  Operator=~=  OutDataTypeStr=boolean  RndMeth=Simplest
  Relational Operator5 : RelationalOperator  Operator===  OutDataTypeStr=boolean  RndMeth=Simplest
  Saturation : Saturate  UpperLimit=TotalTime/Ts  LowerLimit=0  OutDataTypeStr=uint16
  Stop : Subsystem  TreatAsAtomicUnit=on
  Sum : Sum  Inputs=|++  OutDataTypeStr=uint16
  Switch Case : SwitchCase  CaseConditions={1,[2,3]}
  Switch1 : Switch  Criteria=u2 ~= 0  OutDataTypeStr=uint16
  Unit Delay : UnitDelay  SampleTime=-1  HasFrameUpgradeWarning=on
  Unit Delay1 : UnitDelay  SampleTime=-1  HasFrameUpgradeWarning=on
  Unit Delay2 : UnitDelay  SampleTime=-1  HasFrameUpgradeWarning=on
  Omega_ref : Outport
  Vdelta : Outport  Port=2
  wires:
  Constant5/1 -> Sum/1
  Sum/1 -> Saturation/1
  Unit Delay1/1 -> Sum/2
  Saturation/1 -> Switch1/1
  Constant/1 -> Switch1/3
  EN/1 -> Switch1/2
  Switch1/1 -> Add1/1, Relational Operator2/1, Relational Operator1/1, Relational Operator3/1, Unit Delay1/1
  Constant2/1 -> Add1/2, Relational Operator1/2
  Relational Operator1/1 -> Data Type Conversion/1
  Data Type Conversion/1 -> Add/2
  Relational Operator2/1 -> Data Type Conversion1/1
  Data Type Conversion1/1 -> Add/3
  Add/1 -> Relational Operator5/1, Unit Delay2/1, Relational Operator4/1, Switch Case/1  "Mode"
  Merge/1 -> Omega_ref/1
  Merge1/1 -> Vdelta/1
  Constant3/1 -> Relational Operator3/2
  Relational Operator3/1 -> Data Type Conversion2/1
  Data Type Conversion2/1 -> Add/1
  Switch Case/1 -> Lock/Action
  Switch Case/2 -> Accel,VF/Action
  Switch Case/3 -> Stop/Action
  Igamma/1 -> [Igamma]
  Idelta/1 -> [Idelta]
  [Igamma] -> Accel,VF/1(Igamma)  "Igamma"
  [Idelta] -> Lock/1(Idelta), Accel,VF/2(Idelta)  "Idelta"
  Lock/1(Omega_ref) -> Merge/1
  Accel,VF/1(Omega_ref) -> Merge/2
  Stop/1(Omega_ref) -> Merge/3
  Lock/2(Vdelta) -> Merge1/1
  Accel,VF/2(Vdelta) -> Merge1/2
  Stop/2(Vgamma) -> Merge1/3
  Unit Delay/1 -> Accel,VF/4(Vdelta_i)  "Vdelta_i"
  Lock/3(Vdelta_i) -> Unit Delay/1
  Unit Delay2/1 -> Relational Operator4/2  "Vdelta_i"
  Constant1/1 -> Relational Operator5/2
  Relational Operator4/1 -> AND/1  "Mode_Change"
  Relational Operator5/1 -> AND/2  "Mode_Change"
  AND/1 -> Accel,VF/5(Mode_Change)
  Constant6/1 -> Relational Operator2/2
  Add1/1 -> Accel,VF/3(Counter)

== system Vector_Control_Lib/Function-Call Subsystem/簡易センサレス制御/wv_integral ==
  wv_ref : Inport
  Constant : Constant  Value=2*pi  OutDataTypeStr=ufixedTypeTwoPi
  Constant1 : Constant  Value=Ts  OutDataTypeStr=fixedTypeMaxTenThousandth
  Constant3 : Constant  Value=0  OutDataTypeStr=fixdt(1,16)
  Product : Product  OutDataTypeStr=fixedTypeOmegaRefTs
  Relational Operator : RelationalOperator  Operator=<  OutDataTypeStr=boolean  RndMeth=Simplest
  Scope : Scope
  Scope1 : Scope
  Sum : Sum  Inputs=|++  OutDataTypeStr=ufixedTypeTwoPi
  Switch : Switch  Criteria=u2 ~= 0  OutDataTypeStr=ufixedTypeTwoPi
  Unit Delay : UnitDelay  SampleTime=-1  HasFrameUpgradeWarning=on
  Thv : Outport
  wires:
  Product/1 -> Scope/1, Sum/1
  wv_ref/1 -> Product/1
  Relational Operator/1 -> Switch/2
  Sum/1 -> Switch/1, Relational Operator/1
  Constant/1 -> Relational Operator/2
  Switch/1 -> Thv/1, Unit Delay/1
  Unit Delay/1 -> Sum/2
  Constant3/1 -> Switch/3
  Constant1/1 -> Scope1/1, Product/2

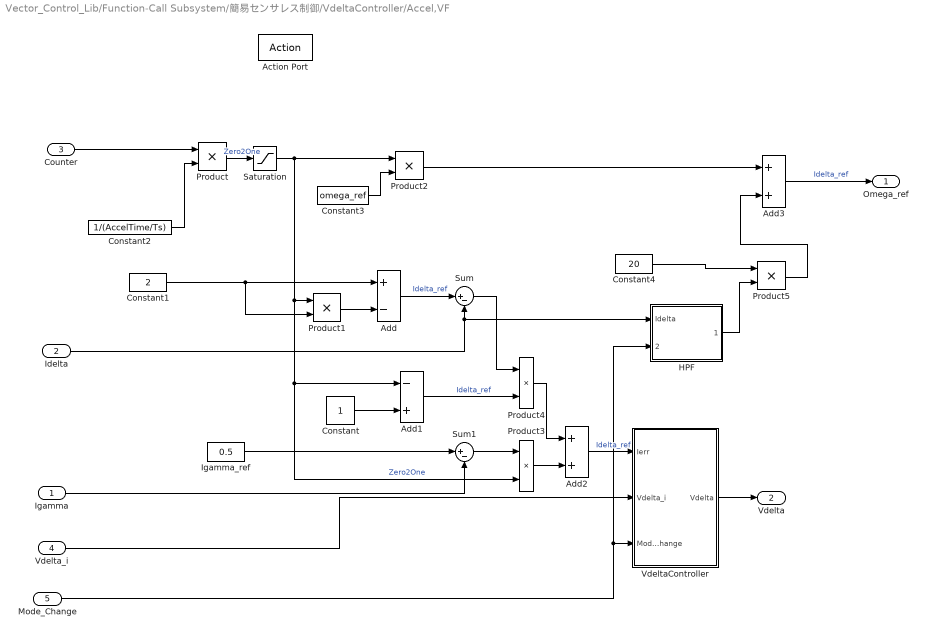
== system Vector_Control_Lib/Function-Call Subsystem/簡易センサレス制御/VdeltaController/Accel,VF ==
  Igamma : Inport
  Idelta : Inport  Port=2
  Counter : Inport  Port=3
  Vdelta_i : Inport  Port=4
  Mode_Change : Inport  Port=5
  Action Port : ActionPort  ActionPortLabel=case [ 2 3 ]:
  Add : Sum  Inputs=+-  OutDataTypeStr=fixdt(1,16,10)
  Add1 : Sum  Inputs=-+  OutDataTypeStr=fixedTypeMaxOne
  Add2 : Sum  OutDataTypeStr=fixdt(1,16,10)
  Add3 : Sum  OutDataTypeStr=fixedTypeOmegaRef
  Constant : Constant  OutDataTypeStr=fixedTypeMaxOne
  Constant1 : Constant  Value=2  OutDataTypeStr=fixdt(1,16,10)
  Constant2 : Constant  Value=1/(AccelTime/Ts)  OutDataTypeStr=fixedTypeMaxTsDivAccelTime
  Constant3 : Constant  Value=omega_ref  OutDataTypeStr=fixedTypeOmegaRef
  Constant4 : Constant  Value=20  OutDataTypeStr=fixdt(1,16,10)
  HPF : Subsystem
  Igamma_ref : Constant  Value=0.5  OutDataTypeStr=fixdt(1,16,10)
  Product : Product  OutDataTypeStr=fixedTypeMaxOne
  Product1 : Product  OutDataTypeStr=fixdt(1,16,10)
  Product{2..5} (4 alike) : Product  OutDataTypeStr=fixedTypeOmegaRef
  Saturation : Saturate  UpperLimit=1  LowerLimit=0  OutDataTypeStr=fixedTypeMaxOne
  Sum : Sum  Inputs=|+-  OutDataTypeStr=fixdt(1,16,10)
  Sum1 : Sum  Inputs=|+-  OutDataTypeStr=fixdt(1,16,10)
  VdeltaController : Subsystem
  Omega_ref : Outport
  Vdelta : Outport  Port=2
  wires:
  Counter/1 -> Product/1
  Constant2/1 -> Product/2
  Product1/1 -> Add/2
  Constant1/1 -> Product1/2, Add/1
  Add/1 -> Sum/1  "Idelta_ref"
  Saturation/1 -> Product2/1, Product1/1, Product3/2, Add1/1  "Zero2One"
  Constant3/1 -> Product2/2
  VdeltaController/1(Vdelta) -> Vdelta/1
  Idelta/1 -> HPF/1(Idelta), Sum/2
  Igamma_ref/1 -> Sum1/1
  Igamma/1 -> Sum1/2
  Sum1/1 -> Product3/1
  Constant/1 -> Add1/2
  Add1/1 -> Product4/2  "Idelta_ref"
  Sum/1 -> Product4/1
  Add2/1 -> VdeltaController/1(Ierr)  "Idelta_ref"
  Product/1 -> Saturation/1  "Zero2One"
  Product4/1 -> Add2/1
  Product3/1 -> Add2/2
  Vdelta_i/1 -> VdeltaController/2(Vdelta_i)
  Mode_Change/1 -> HPF/2(Mode_Change), VdeltaController/3(Mode_Change)
  Add3/1 -> Omega_ref/1  "Idelta_ref"
  Product2/1 -> Add3/1
  HPF/1(Idelta_hpf) -> Product5/2
  Constant4/1 -> Product5/1
  Product5/1 -> Add3/2

== system Vector_Control_Lib/Function-Call Subsystem/簡易センサレス制御/VdeltaController/Lock ==
  Idelta : Inport
  Action Port : ActionPort  ActionPortLabel=case [ 1 ]:
  Constant : Constant  Value=0  OutDataTypeStr=fixedTypeOmegaRef
  Constant1 : Constant  Value=2  OutDataTypeStr=fixdt(1,16,10)
  VdeltaController : Subsystem
  Omega_ref : Outport
  Vdelta : Outport  Port=2
  Vdelta_i : Outport  Port=3
  wires:
  Constant/1 -> Omega_ref/1
  Constant1/1 -> VdeltaController/1(Idelta_ref)
  VdeltaController/1(Vdelta) -> Vdelta/1
  Idelta/1 -> VdeltaController/2(Idelta)
  VdeltaController/2(Vdelta_i) -> Vdelta_i/1

== system Vector_Control_Lib/Function-Call Subsystem/簡易センサレス制御/VdeltaController/Stop ==
  Action Port : ActionPort  ActionPortLabel=default:
  Constant : Constant  Value=0  OutDataTypeStr=fixedTypeOmegaRef
  Constant1 : Constant  Value=0  OutDataTypeStr=fixdt(1,16,10)
  Omega_ref : Outport
  Vgamma : Outport  Port=2
  wires:
  Constant1/1 -> Vgamma/1
  Constant/1 -> Omega_ref/1

== system Vector_Control_Lib/Function-Call Subsystem/簡易センサレス制御/VdeltaController/Accel,VF/HPF ==
  Idelta : Inport
  Mode_Change : Inport  Port=2
  Add : Sum  Inputs=+-  OutDataTypeStr=fixdt(1,16,10)
  Constant1 : Constant  Value=k_LPF  OutDataTypeStr=fixedTypeMaxOne
  Constant2 : Constant  Value=1-k_LPF  OutDataTypeStr=fixedTypeMaxOne
  Product1 : Product  OutDataTypeStr=fixdt(1,32,26)
  Product2 : Product  OutDataTypeStr=fixdt(1,32,26)
  Scope : Scope  NumInputPorts=3
  Sum1 : Sum  Inputs=|++  OutDataTypeStr=fixdt(1,32,26)
  Switch : Switch  Criteria=u2 ~= 0
  Unit Delay : UnitDelay  SampleTime=-1  HasFrameUpgradeWarning=on
  Idelta_hpf : Outport
  wires:
  Constant1/1 -> Product1/2
  Sum1/1 -> Scope/2, Add/2, Unit Delay/1
  Unit Delay/1 -> Switch/3
  Mode_Change/1 -> Switch/2
  Switch/1 -> Product1/1
  Product1/1 -> Sum1/2
  Constant2/1 -> Product2/2
  Idelta/1 -> Scope/1, Add/1, Switch/1, Product2/1
  Product2/1 -> Sum1/1
  Add/1 -> Scope/3, Idelta_hpf/1

== system Vector_Control_Lib/Function-Call Subsystem/簡易センサレス制御/VdeltaController/Accel,VF/VdeltaController ==
  Ierr : Inport
  Vdelta_i : Inport  Port=2
  Mode_Change : Inport  Port=3
  Add : Sum  OutDataTypeStr=fixdt(1,16,10)
  Constant : Constant  Value=Kp  OutDataTypeStr=fixdt(1,16,16)
  Constant1 : Constant  Value=Ki_Ts  OutDataTypeStr=fixdt(1,16)
  Product : Product  OutDataTypeStr=fixdt(1,16,10)
  Product1 : Product  OutDataTypeStr=fixdt(1,32,26)
  Saturation : Saturate  UpperLimit=31  LowerLimit=-31  OutDataTypeStr=fixdt(1,16,10)
  Sum1 : Sum  Inputs=|++  OutDataTypeStr=fixdt(1,32,26)
  Switch : Switch  Criteria=u2 ~= 0
  Unit Delay : UnitDelay  SampleTime=-1  HasFrameUpgradeWarning=on
  Vdelta : Outport
  wires:
  Ierr/1 -> Product1/1, Product/1
  Constant/1 -> Product/2
  Constant1/1 -> Product1/2
  Product1/1 -> Sum1/1
  Sum1/1 -> Saturation/1, Unit Delay/1
  Product/1 -> Add/1
  Add/1 -> Vdelta/1
  Saturation/1 -> Add/2
  Switch/1 -> Sum1/2
  Vdelta_i/1 -> Switch/1
  Unit Delay/1 -> Switch/3
  Mode_Change/1 -> Switch/2

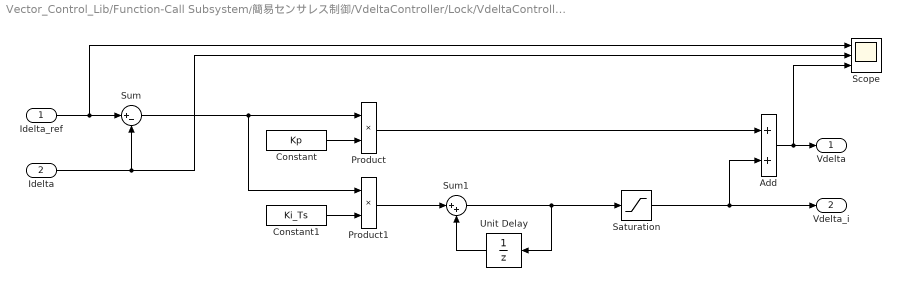
== system Vector_Control_Lib/Function-Call Subsystem/簡易センサレス制御/VdeltaController/Lock/VdeltaController ==
  Idelta_ref : Inport
  Idelta : Inport  Port=2
  Add : Sum  OutDataTypeStr=fixdt(1,16,10)
  Constant : Constant  Value=Kp  OutDataTypeStr=fixdt(1,16,16)
  Constant1 : Constant  Value=Ki_Ts  OutDataTypeStr=fixdt(1,16)
  Product : Product  OutDataTypeStr=fixdt(1,16,10)
  Product1 : Product  OutDataTypeStr=fixdt(1,32,26)
  Saturation : Saturate  UpperLimit=31  LowerLimit=-31  OutDataTypeStr=fixdt(1,16,10)
  Scope : Scope  NumInputPorts=3
  Sum : Sum  Inputs=|+-
  Sum1 : Sum  Inputs=|++  OutDataTypeStr=fixdt(1,32,26)
  Unit Delay : UnitDelay  SampleTime=-1  HasFrameUpgradeWarning=on
  Vdelta : Outport
  Vdelta_i : Outport  Port=2
  wires:
  Idelta_ref/1 -> Scope/1, Sum/1
  Idelta/1 -> Scope/2, Sum/2
  Sum/1 -> Product1/1, Product/1
  Constant/1 -> Product/2
  Constant1/1 -> Product1/2
  Product1/1 -> Sum1/1
  Unit Delay/1 -> Sum1/2
  Sum1/1 -> Saturation/1, Unit Delay/1
  Product/1 -> Add/1
  Add/1 -> Scope/3, Vdelta/1
  Saturation/1 -> Add/2, Vdelta_i/1
